simulink model "untitled"  (R2020b)
settings: Solver=VariableStepAuto  StartTime=0.0  StopTime=10.0  RelTol=1e-3
values from neighbouring files (symbols this model uses):
  c1 = 1.2801    [input.m]
  c2 = 23.99    [input.m]
  c3 = 0.52    [input.m]
  c4 = 0.03    [input.m]
  fn = m*9.81    (= 3355.02)    [input.m]
  jw = 1.13    [input.m]
  m = 342    [input.m]
  r = 0.33    [input.m]
settings Model: Creator=K E S SRINIVAS  LastModifiedBy=K E S SRINIVAS

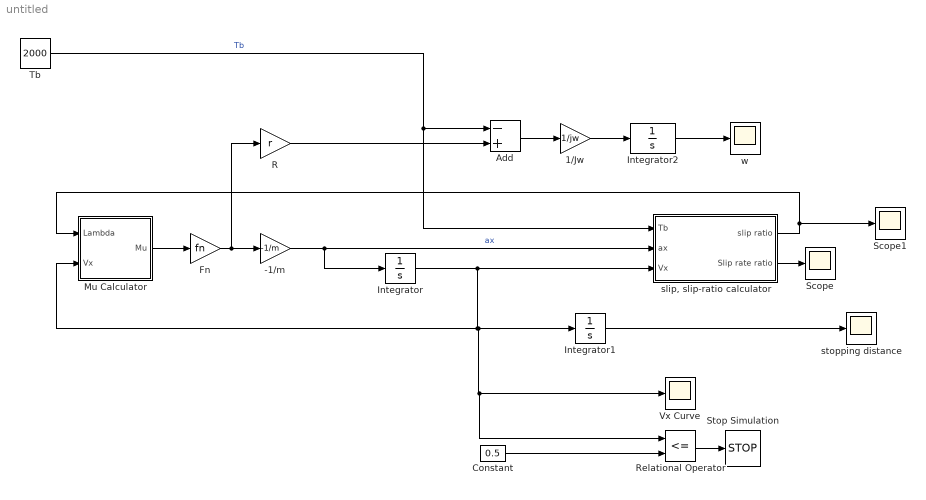
== system untitled ==
  -1/m : Gain  Gain=-1/m
  1/Jw : Gain  Gain=1/jw
  Add : Sum  Inputs=-+
  Constant : Constant  Value=0.5
  Fn : Gain  Gain=fn
  Integrator : Integrator
  Integrator1 : Integrator
  Integrator2 : Integrator
  Mu Calculator : Subsystem
  R : Gain  Gain=r
  Relational Operator : RelationalOperator  Operator=<=  OutDataTypeStr=boolean  RndMeth=Simplest
  Scope : Scope
  Scope1 : Scope
  Stop Simulation : Stop
  Tb : Constant  Value=2000
  Vx Curve : Scope
  "slip, slip-ratio calculator" : Subsystem
  stopping distance : Scope
  w : Scope
  wires:
  Tb/1 -> Add/1, "slip, slip-ratio calculator"/1(Tb)  "Tb"
  Integrator/1 -> Mu Calculator/2(Vx), Relational Operator/1, Vx Curve/1, Integrator1/1, "slip, slip-ratio calculator"/3(Vx)
  -1/m/1 -> Integrator/1, "slip, slip-ratio calculator"/2(ax)  "ax"
  Integrator1/1 -> stopping distance/1
  Constant/1 -> Relational Operator/2
  Relational Operator/1 -> Stop Simulation/1
  "slip, slip-ratio calculator"/1(slip ratio) -> Scope1/1, Mu Calculator/1(Lambda)
  Mu Calculator/1(Mu) -> Fn/1
  Fn/1 -> R/1, -1/m/1
  R/1 -> Add/2
  Add/1 -> 1/Jw/1
  1/Jw/1 -> Integrator2/1
  Integrator2/1 -> w/1
  "slip, slip-ratio calculator"/2(Slip rate ratio) -> Scope/1

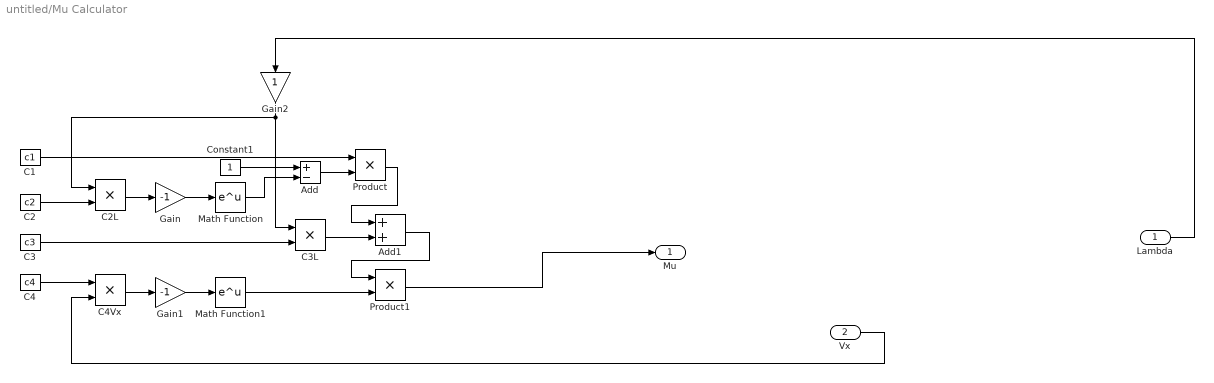
== system untitled/Mu Calculator ==
  Lambda : Inport
  Vx : Inport  Port=2
  Add : Sum  Inputs=+-
  Add1 : Sum
  C1 : Constant  Value=c1
  C2 : Constant  Value=c2
  C2L : Product
  C3 : Constant  Value=c3
  C3L : Product
  C4 : Constant  Value=c4
  C4Vx : Product
  Constant1 : Constant
  Gain : Gain  Gain=-1
  Gain1 : Gain  Gain=-1
  Gain2 : Gain
  Math Function : Math  SaturateOnIntegerOverflow=on
  Math Function1 : Math  SaturateOnIntegerOverflow=on
  Product : Product
  Product1 : Product
  Mu : Outport
  wires:
  C2/1 -> C2L/2
  Gain/1 -> Math Function/1
  C1/1 -> Product/1
  C2L/1 -> Gain/1
  Constant1/1 -> Add/1
  Vx/1 -> C4Vx/2
  C4/1 -> C4Vx/1
  Add/1 -> Product/2
  Math Function/1 -> Add/2
  Gain1/1 -> Math Function1/1
  Math Function1/1 -> Product1/2
  C3L/1 -> Add1/2
  Gain2/1 -> C3L/1, C2L/1
  Product1/1 -> Mu/1
  C4Vx/1 -> Gain1/1
  C3/1 -> C3L/2
  Product/1 -> Add1/1
  Add1/1 -> Product1/1
  Lambda/1 -> Gain2/1

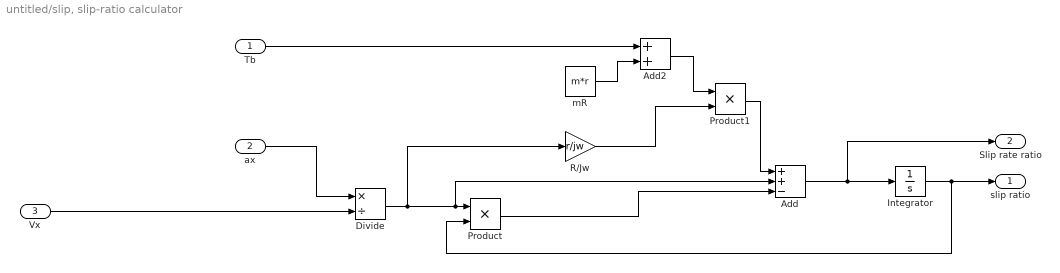
== system untitled/slip, slip-ratio calculator ==
  Tb : Inport
  ax : Inport  Port=2
  Vx : Inport  Port=3
  Add : Sum  Inputs=++-
  Add2 : Sum
  Divide : Product  Inputs=*/
  Integrator : Integrator
  Product : Product
  Product1 : Product
  R/Jw : Gain  Gain=r/jw
  mR : Constant  Value=m*r
  slip ratio : Outport
  Slip rate ratio : Outport  Port=2
  wires:
  ax/1 -> Divide/1
  Divide/1 -> R/Jw/1, Add/2, Product/1
  Product1/1 -> Add/1
  Add2/1 -> Product1/1
  Product/1 -> Add/3
  Add/1 -> Slip rate ratio/1, Integrator/1
  mR/1 -> Add2/2
  R/Jw/1 -> Product1/2
  Tb/1 -> Add2/1
  Integrator/1 -> Product/2, slip ratio/1
  Vx/1 -> Divide/2
